simulink library "VIS_LIB"  (Simulink 8.6)
settings: Solver=ode45  StartTime=0.0  StopTime=10.0  RelTol=1e-3
undefined symbols (not defined in the file): AC, SIXOSEM_F_WD_AC_MASTER
libraries: cdsFilt x376, cdsEpicsOut x253, cdsEpicsIn x179, cdsTP x123, VIS_LIB x95, cdsMuxMatrix x91, cdsEpicsStringIn x75, cdsFiltCtrl x72, cdsFunctionCall x70, cdsRms x59, KAGRA_UTIL x25, STATE_BIO_MASTER x5
(part 6 of 38)

== system VIS_LIB/PReQua_3DOF ==
  Freq : Inport
  t : Inport  Port=2
  SampFreq : Inport  Port=3
  LEN_SIG : Inport  Port=4
  PIT_SIG : Inport  Port=5
  YAW_SIG1 : Inport  Port=6
  LEN_PHASE : Inport  Port=7
  PIT_PHASE : Inport  Port=8
  YAW_PHASE1 : Inport  Port=9
  Demux{1..6} (6 alike) : Demux  Outputs=3
  ENV_LEN : cdsFilt/Subsystem  Tag=cdsFilt  Description=|
      | Purpose:                                                                                                                                                                                                                                  
      | Standard CDS IIR filter module.                                                                                                                                                                                                           
      |                                                                                                                                                                                                                                           
      | Operation:                                                                                                                                                                                                                                
      | Consists of 10 second order section IIR filters, plus a ramped gain stage. In FE code, also provides pre-defined test points and excitation channel inputs. The filter coefficients are defined in the LIGO system using the 'foton' tool.
      |                                                                                                                                                                                                                                           
      | Usage:                                                                                                                                                                                                                                    
      | Name the part with the desired filter module name.
      settings: AttributesFormatString=%<Tag>
  ENV_PIT : cdsFilt/Subsystem  Tag=cdsFilt  Description=|
      | Purpose:                                                                                                                                                                                                                                  
      | Standard CDS IIR filter module.                                                                                                                                                                                                           
      |                                                                                                                                                                                                                                           
      | Operation:                                                                                                                                                                                                                                
      | Consists of 10 second order section IIR filters, plus a ramped gain stage. In FE code, also provides pre-defined test points and excitation channel inputs. The filter coefficients are defined in the LIGO system using the 'foton' tool.
      |                                                                                                                                                                                                                                           
      | Usage:                                                                                                                                                                                                                                    
      | Name the part with the desired filter module name.
      settings: AttributesFormatString=%<Tag>
  ENV_YAW : cdsFilt/Subsystem  Tag=cdsFilt  Description=|
      | Purpose:                                                                                                                                                                                                                                  
      | Standard CDS IIR filter module.                                                                                                                                                                                                           
      |                                                                                                                                                                                                                                           
      | Operation:                                                                                                                                                                                                                                
      | Consists of 10 second order section IIR filters, plus a ramped gain stage. In FE code, also provides pre-defined test points and excitation channel inputs. The filter coefficients are defined in the LIGO system using the 'foton' tool.
      |                                                                                                                                                                                                                                           
      | Usage:                                                                                                                                                                                                                                    
      | Name the part with the desired filter module name.
      settings: AttributesFormatString=%<Tag>
  LEN_CP : VIS_LIB/CALC_CP_COEF_3DOF
  Mux1 : Mux  Inputs=3
  Mux4 : Mux  Inputs=3
  PIT_CP : VIS_LIB/CALC_CP_COEF_3DOF
  QUALEN : KAGRA_UTIL/pReQua_ver2
  QUAPIT : KAGRA_UTIL/pReQua_ver2
  QUAYAW : KAGRA_UTIL/pReQua_ver2
  YAW_CP : VIS_LIB/CALC_CP_COEF_3DOF
  PhaseL : Outport
  PhaseP : Outport  Port=2
  PhaseY : Outport  Port=3
  wires:
  QUAPIT/1 -> ENV_PIT/1
  QUAPIT/2 -> PhaseP/1
  QUAYAW/1 -> ENV_YAW/1
  QUAYAW/2 -> PhaseY/1
  LEN_SIG/1 -> QUALEN/1
  LEN_PHASE/1 -> QUALEN/2
  PIT_SIG/1 -> QUAPIT/1
  PIT_PHASE/1 -> QUAPIT/2
  YAW_SIG1/1 -> QUAYAW/1
  YAW_PHASE1/1 -> QUAYAW/2
  Freq/1 -> Mux4/1
  t/1 -> Mux4/2
  SampFreq/1 -> Mux4/3
  Demux1/1 -> QUAPIT/3
  Demux1/2 -> QUAPIT/4
  Demux1/3 -> QUAPIT/5
  Demux2/1 -> QUAYAW/3
  Demux2/2 -> QUAYAW/4
  Demux2/3 -> QUAYAW/5
  Mux4/1 -> Demux1/1, Demux2/1, Demux6/1
  ENV_LEN/1 -> Mux1/1
  ENV_PIT/1 -> Mux1/2
  ENV_YAW/1 -> Mux1/3
  Demux3/2 -> LEN_CP/3
  Demux3/1 -> LEN_CP/1, LEN_CP/2
  Demux3/3 -> LEN_CP/4
  Demux4/1 -> PIT_CP/2
  Demux4/2 -> PIT_CP/1, PIT_CP/3
  Demux4/3 -> PIT_CP/4
  Demux5/1 -> YAW_CP/2
  Demux5/2 -> YAW_CP/3
  Demux5/3 -> YAW_CP/1, YAW_CP/4
  Mux1/1 -> Demux5/1, Demux4/1, Demux3/1
  Demux6/1 -> QUALEN/3
  Demux6/2 -> QUALEN/4
  Demux6/3 -> QUALEN/5
  QUALEN/2 -> PhaseL/1
  QUALEN/1 -> ENV_LEN/1

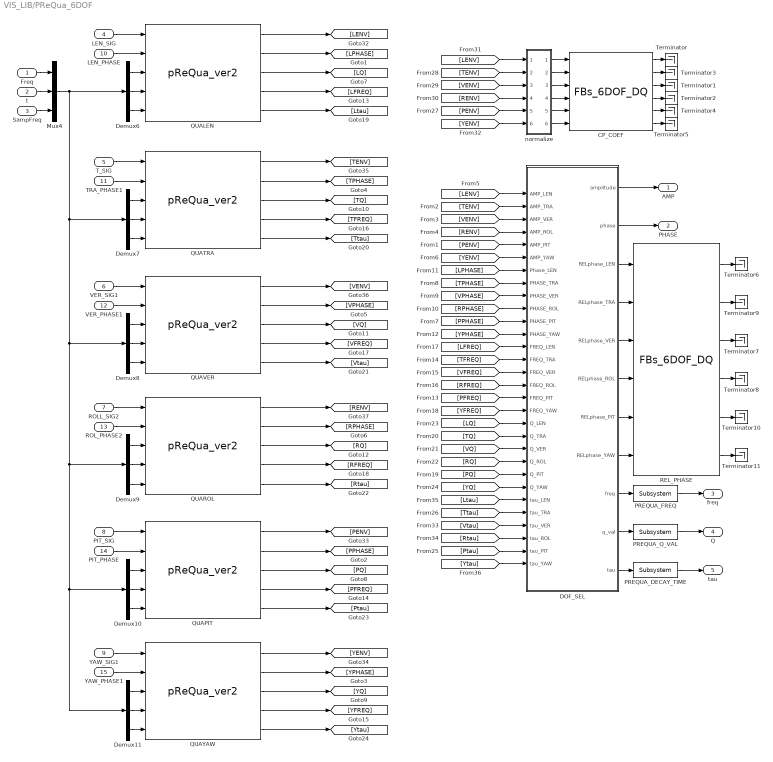
== system VIS_LIB/PReQua_6DOF ==
  Freq : Inport
  t : Inport  Port=2
  SampFreq : Inport  Port=3
  LEN_SIG : Inport  Port=4
  T_SIG : Inport  Port=5
  VER_SIG1 : Inport  Port=6
  ROLL_SIG2 : Inport  Port=7
  PIT_SIG : Inport  Port=8
  YAW_SIG1 : Inport  Port=9
  LEN_PHASE : Inport  Port=10
  TRA_PHASE1 : Inport  Port=11
  VER_PHASE1 : Inport  Port=12
  ROL_PHASE2 : Inport  Port=13
  PIT_PHASE : Inport  Port=14
  YAW_PHASE1 : Inport  Port=15
  CP_COEF : VIS_LIB/UTILs/FBs_6DOF_DQ
  DOF_SEL : Subsystem
  Demux{6..11} (6 alike) : Demux  Outputs=3
  Mux4 : Mux  Inputs=3
  PREQUA_DECAY_TIME : cdsFilt/Subsystem  Tag=cdsFilt  Description=|
      | Purpose:                                                                                                                                                                                                                                  
      | Standard CDS IIR filter module.                                                                                                                                                                                                           
      |                                                                                                                                                                                                                                           
      | Operation:                                                                                                                                                                                                                                
      | Consists of 10 second order section IIR filters, plus a ramped gain stage. In FE code, also provides pre-defined test points and excitation channel inputs. The filter coefficients are defined in the LIGO system using the 'foton' tool.
      |                                                                                                                                                                                                                                           
      | Usage:                                                                                                                                                                                                                                    
      | Name the part with the desired filter module name.
      settings: AttributesFormatString=%<Tag>
  PREQUA_FREQ : cdsFilt/Subsystem  Tag=cdsFilt  Description=|
      | Purpose:                                                                                                                                                                                                                                  
      | Standard CDS IIR filter module.                                                                                                                                                                                                           
      |                                                                                                                                                                                                                                           
      | Operation:                                                                                                                                                                                                                                
      | Consists of 10 second order section IIR filters, plus a ramped gain stage. In FE code, also provides pre-defined test points and excitation channel inputs. The filter coefficients are defined in the LIGO system using the 'foton' tool.
      |                                                                                                                                                                                                                                           
      | Usage:                                                                                                                                                                                                                                    
      | Name the part with the desired filter module name.
      settings: AttributesFormatString=%<Tag>
  PREQUA_Q_VAL : cdsFilt/Subsystem  Tag=cdsFilt  Description=|
      | Purpose:                                                                                                                                                                                                                                  
      | Standard CDS IIR filter module.                                                                                                                                                                                                           
      |                                                                                                                                                                                                                                           
      | Operation:                                                                                                                                                                                                                                
      | Consists of 10 second order section IIR filters, plus a ramped gain stage. In FE code, also provides pre-defined test points and excitation channel inputs. The filter coefficients are defined in the LIGO system using the 'foton' tool.
      |                                                                                                                                                                                                                                           
      | Usage:                                                                                                                                                                                                                                    
      | Name the part with the desired filter module name.
      settings: AttributesFormatString=%<Tag>
  QUALEN : KAGRA_UTIL/pReQua_ver2
  QUAPIT : KAGRA_UTIL/pReQua_ver2
  QUAROL : KAGRA_UTIL/pReQua_ver2
  QUATRA : KAGRA_UTIL/pReQua_ver2
  QUAVER : KAGRA_UTIL/pReQua_ver2
  QUAYAW : KAGRA_UTIL/pReQua_ver2
  REL_PHASE : VIS_LIB/UTILs/FBs_6DOF_DQ
  Terminator{,1..11} (12 alike) : Terminator
  normalize : Subsystem
  AMP : Outport
  PHASE : Outport  Port=2
  freq : Outport  Port=3
  Q : Outport  Port=4
  tau : Outport  Port=5
  wires:
  DOF_SEL/8(RELphase_YAW) -> REL_PHASE/6
  DOF_SEL/7(RELphase_PIT) -> REL_PHASE/5
  DOF_SEL/6(RELphase_ROL) -> REL_PHASE/4
  DOF_SEL/5(RELphase_VER) -> REL_PHASE/3
  DOF_SEL/4(RELphase_TRA) -> REL_PHASE/2
  DOF_SEL/3(RELphase_LEN) -> REL_PHASE/1
  PREQUA_DECAY_TIME/1 -> tau/1
  PREQUA_Q_VAL/1 -> Q/1
  PREQUA_FREQ/1 -> freq/1
  REL_PHASE/6 -> Terminator11/1
  REL_PHASE/5 -> Terminator10/1
  REL_PHASE/4 -> Terminator8/1
  REL_PHASE/3 -> Terminator7/1
  REL_PHASE/2 -> Terminator9/1
  REL_PHASE/1 -> Terminator6/1
  CP_COEF/6 -> Terminator5/1
  CP_COEF/5 -> Terminator4/1
  CP_COEF/4 -> Terminator2/1
  CP_COEF/3 -> Terminator1/1
  normalize/6(Out6) -> CP_COEF/6
  normalize/5(Out5) -> CP_COEF/5
  normalize/4(Out4) -> CP_COEF/4
  normalize/3(Out3) -> CP_COEF/3
  normalize/2(Out2) -> CP_COEF/2
  normalize/1(Out1) -> CP_COEF/1
  [Ytau] -> DOF_SEL/30(tau_YAW)
  [Ptau] -> DOF_SEL/29(tau_PIT)
  [Rtau] -> DOF_SEL/28(tau_ROL)
  [Vtau] -> DOF_SEL/27(tau_VER)
  [Ttau] -> DOF_SEL/26(tau_TRA)
  [Ltau] -> DOF_SEL/25(tau_LEN)
  DOF_SEL/11(tau) -> PREQUA_DECAY_TIME/1
  QUAPIT/5 -> [Ptau]
  QUAYAW/5 -> [Ytau]
  QUAVER/5 -> [Vtau]
  QUAROL/5 -> [Rtau]
  QUATRA/5 -> [Ttau]
  QUALEN/5 -> [Ltau]
  DOF_SEL/10(q_val) -> PREQUA_Q_VAL/1
  DOF_SEL/9(freq) -> PREQUA_FREQ/1
  QUALEN/4 -> [LFREQ]
  QUAPIT/4 -> [PFREQ]
  QUAYAW/4 -> [YFREQ]
  QUATRA/4 -> [TFREQ]
  QUAVER/4 -> [VFREQ]
  QUAROL/4 -> [RFREQ]
  QUALEN/3 -> [LQ]
  QUAPIT/3 -> [PQ]
  QUAYAW/3 -> [YQ]
  QUATRA/3 -> [TQ]
  QUAVER/3 -> [VQ]
  QUAROL/3 -> [RQ]
  [YQ] -> DOF_SEL/24(Q_YAW)
  [PQ] -> DOF_SEL/23(Q_PIT)
  [RQ] -> DOF_SEL/22(Q_ROL)
  [VQ] -> DOF_SEL/21(Q_VER)
  [TQ] -> DOF_SEL/20(Q_TRA)
  [LQ] -> DOF_SEL/19(Q_LEN)
  [YFREQ] -> DOF_SEL/18(FREQ_YAW)
  [PFREQ] -> DOF_SEL/17(FREQ_PIT)
  [RFREQ] -> DOF_SEL/16(FREQ_ROL)
  [VFREQ] -> DOF_SEL/15(FREQ_VER)
  [TFREQ] -> DOF_SEL/14(FREQ_TRA)
  [LFREQ] -> DOF_SEL/13(FREQ_LEN)
  DOF_SEL/2(phase) -> PHASE/1
  DOF_SEL/1(amplitude) -> AMP/1
  [YPHASE] -> DOF_SEL/12(PHASE_YAW)
  [PPHASE] -> DOF_SEL/11(PHASE_PIT)
  [RPHASE] -> DOF_SEL/10(PHASE_ROL)
  [VPHASE] -> DOF_SEL/9(PHASE_VER)
  [TPHASE] -> DOF_SEL/8(PHASE_TRA)
  [LPHASE] -> DOF_SEL/7(Phase_LEN)
  [YENV] -> DOF_SEL/6(AMP_YAW)
  [PENV] -> DOF_SEL/5(AMP_PIT)
  [RENV] -> DOF_SEL/4(AMP_ROL)
  [VENV] -> DOF_SEL/3(AMP_VER)
  [TENV] -> DOF_SEL/2(AMP_TRA)
  [LENV] -> DOF_SEL/1(AMP_LEN)
  QUALEN/2 -> [LPHASE]
  CP_COEF/2 -> Terminator3/1
  CP_COEF/1 -> Terminator/1
  QUAPIT/2 -> [PPHASE]
  QUAYAW/2 -> [YPHASE]
  QUAVER/2 -> [VPHASE]
  QUATRA/2 -> [TPHASE]
  QUAROL/2 -> [RPHASE]
  QUALEN/1 -> [LENV]
  QUAPIT/1 -> [PENV]
  QUAYAW/1 -> [YENV]
  QUATRA/1 -> [TENV]
  QUAVER/1 -> [VENV]
  QUAROL/1 -> [RENV]
  LEN_SIG/1 -> QUALEN/1
  LEN_PHASE/1 -> QUALEN/2
  T_SIG/1 -> QUATRA/1
  VER_SIG1/1 -> QUAVER/1
  YAW_SIG1/1 -> QUAYAW/1
  PIT_SIG/1 -> QUAPIT/1
  ROLL_SIG2/1 -> QUAROL/1
  YAW_PHASE1/1 -> QUAYAW/2
  PIT_PHASE/1 -> QUAPIT/2
  ROL_PHASE2/1 -> QUAROL/2
  VER_PHASE1/1 -> QUAVER/2
  TRA_PHASE1/1 -> QUATRA/2
  Demux6/1 -> QUALEN/3
  Demux6/2 -> QUALEN/4
  Demux6/3 -> QUALEN/5
  Freq/1 -> Mux4/1
  t/1 -> Mux4/2
  SampFreq/1 -> Mux4/3
  Demux7/1 -> QUATRA/3
  Demux7/2 -> QUATRA/4
  Demux7/3 -> QUATRA/5
  Demux8/1 -> QUAVER/3
  Demux8/2 -> QUAVER/4
  Demux8/3 -> QUAVER/5
  Demux9/1 -> QUAROL/3
  Demux9/2 -> QUAROL/4
  Demux9/3 -> QUAROL/5
  Demux10/1 -> QUAPIT/3
  Demux10/2 -> QUAPIT/4
  Demux10/3 -> QUAPIT/5
  Demux11/1 -> QUAYAW/3
  Demux11/2 -> QUAYAW/4
  Demux11/3 -> QUAYAW/5
  Mux4/1 -> Demux7/1, Demux8/1, Demux10/1, Demux11/1, Demux9/1, Demux6/1
  [LENV] -> normalize/1(In1)
  [TENV] -> normalize/2(In2)
  [VENV] -> normalize/3(In3)
  [RENV] -> normalize/4(In4)
  [PENV] -> normalize/5(In5)
  [YENV] -> normalize/6(In6)

== system VIS_LIB/QUAASC1 ==
  Freq : Inport
  t : Inport  Port=2
  SampFreq : Inport  Port=3
  P_SIG : Inport  Port=4
  Y_SIG : Inport  Port=5
  P_SIG2 : Inport  Port=6
  Y_SIG2 : Inport  Port=7
  P_PHASE1 : Inport  Port=8
  Y_PHASE1 : Inport  Port=9
  P_PHASE2 : Inport  Port=10
  Y_PHASE2 : Inport  Port=11
  CP_COEF : Subsystem
  DOF_SEL : Subsystem
  Demux{6..9} (4 alike) : Demux  Outputs=3
  ETM_PIT : KAGRA_UTIL/pReQua_ver2
  ETM_YAW : KAGRA_UTIL/pReQua_ver2
  ITM_PIT : KAGRA_UTIL/pReQua_ver2
  ITM_YAW : KAGRA_UTIL/pReQua_ver2
  Mux4 : Mux  Inputs=3
  REL_PHASE : Subsystem
  Terminator{,1..19} (20 alike) : Terminator
  normalize : Subsystem
  wires:
  CP_COEF/4(ROL_OUT) -> Terminator2/1
  CP_COEF/3(VER_OUT) -> Terminator1/1
  normalize/4(Out4) -> CP_COEF/4(ROL_IN)
  normalize/3(Out3) -> CP_COEF/3(VER_IN)
  normalize/2(Out2) -> CP_COEF/2(TRA_IN)
  normalize/1(Out1) -> CP_COEF/1(LEN_IN)
  CP_COEF/2(TRA_OUT) -> Terminator3/1
  CP_COEF/1(LEN_OUT) -> Terminator/1
  ITM_PIT/1 -> [ENVITMP]
  ITM_YAW/1 -> [ENVITMY]
  ETM_PIT/1 -> [ENVETMP]
  ETM_YAW/1 -> [ENVETMY]
  P_SIG/1 -> ITM_PIT/1
  P_PHASE1/1 -> ITM_PIT/2
  Y_SIG/1 -> ITM_YAW/1
  P_SIG2/1 -> ETM_PIT/1
  Y_SIG2/1 -> ETM_YAW/1
  Y_PHASE2/1 -> ETM_YAW/2
  P_PHASE2/1 -> ETM_PIT/2
  Y_PHASE1/1 -> ITM_YAW/2
  Demux6/1 -> ITM_PIT/3
  Demux6/2 -> ITM_PIT/4
  Demux6/3 -> ITM_PIT/5
  Freq/1 -> Mux4/1
  t/1 -> Mux4/2
  SampFreq/1 -> Mux4/3
  Demux7/1 -> ITM_YAW/3
  Demux7/2 -> ITM_YAW/4
  Demux7/3 -> ITM_YAW/5
  Demux8/1 -> ETM_PIT/3
  Demux8/2 -> ETM_PIT/4
  Demux8/3 -> ETM_PIT/5
  Demux9/1 -> ETM_YAW/3
  Demux9/2 -> ETM_YAW/4
  Demux9/3 -> ETM_YAW/5
  Mux4/1 -> Demux7/1, Demux8/1, Demux9/1, Demux6/1
  ITM_PIT/5 -> Terminator4/1
  ITM_PIT/4 -> Terminator5/1
  ITM_PIT/3 -> Terminator6/1
  ITM_YAW/5 -> Terminator8/1
  ITM_YAW/4 -> Terminator9/1
  ITM_YAW/3 -> Terminator10/1
  ETM_PIT/5 -> Terminator12/1
  ETM_PIT/4 -> Terminator13/1
  ETM_PIT/3 -> Terminator14/1
  ETM_YAW/5 -> Terminator16/1
  ETM_YAW/4 -> Terminator17/1
  ETM_YAW/3 -> Terminator18/1
  ITM_PIT/2 -> [PHITMP]
  ITM_YAW/2 -> [PHITMY]
  ETM_PIT/2 -> [PHETMP]
  ETM_YAW/2 -> [PHETMY]
  [ENVITMP] -> normalize/1(In1)
  [ENVITMY] -> normalize/2(In2)
  [ENVETMP] -> normalize/3(In3)
  [ENVETMY] -> normalize/4(In4)
  [PHITMP] -> DOF_SEL/1(Phase_LEN)
  [PHITMY] -> DOF_SEL/2(PHASE_TRA)
  [PHETMP] -> DOF_SEL/3(PHASE_VER)
  [PHETMY] -> DOF_SEL/4(PHASE_ROL)
  DOF_SEL/1(RELphase_LEN) -> REL_PHASE/1(LEN_IN)
  DOF_SEL/2(RELphase_TRA) -> REL_PHASE/2(TRA_IN)
  DOF_SEL/3(RELphase_VER) -> REL_PHASE/3(VER_IN)
  DOF_SEL/4(RELphase_ROL) -> REL_PHASE/4(ROL_IN)
  REL_PHASE/4(ROL_OUT) -> Terminator15/1
  REL_PHASE/3(VER_OUT) -> Terminator11/1
  REL_PHASE/2(TRA_OUT) -> Terminator19/1
  REL_PHASE/1(LEN_OUT) -> Terminator7/1

== system VIS_LIB/SHUTDOWN_TRIG_TYPEBP ==
  note: WDBLOCKFLAG is zero (0) if OK,
      | non-zero if BAD
  note: AND is zero  (0) if all stages are OK
      | non-zero if BAD
  SF_WDBLOCKFLAG_In : Inport
  BF_WDBLOCKFLAG_In : Inport  Port=2
  IM_WDBLOCKFLAG_In : Inport  Port=3
  TM_WDBLOCKFLAG_In : Inport  Port=4
  LogicalOperator1 : Logic  Operator=OR  Inputs=4  AllPortsSameDT=off  OutDataTypeStr=boolean
  STATE : cdsEpicsOut/Subsystem  Tag=cdsEpicsOutput  Description=|
      | Purpose:                                          
      | Output a FE signal to an EPICS channel.           
      |                                                   
      | Operation:                                        
      | Takes input value and passes it to EPICS record.  
      |                                                   
      | Usage:                                            
      | Name the part with the desired EPICS rrecord name.
      settings: AttributesFormatString=%<Tag>
  DACKILL_TRIG_Out : Outport
  wires:
  STATE/1 -> DACKILL_TRIG_Out/1
  LogicalOperator1/1 -> STATE/1
  SF_WDBLOCKFLAG_In/1 -> LogicalOperator1/1
  BF_WDBLOCKFLAG_In/1 -> LogicalOperator1/2
  IM_WDBLOCKFLAG_In/1 -> LogicalOperator1/3
  TM_WDBLOCKFLAG_In/1 -> LogicalOperator1/4

== system VIS_LIB/UTILs ==
  1COIL_DQ : Subsystem
  3COILs : Subsystem
  3COILs_DQ : Subsystem
  4COILs : Subsystem
  4COILs_DQ : Subsystem
  4SEG_DQ : Subsystem
  6COILs : Subsystem
  6COILs_DQ : Subsystem
  7COILs_DQ1 : Subsystem
  DRIVEALIGN : Subsystem
  FBs_2DOF : Subsystem
  FBs_2DOF_DQ : Subsystem
  FBs_3DOF : Subsystem
  FBs_3DOF_DQ : Subsystem
  FBs_3DOF_IP : Subsystem
  FBs_3DOF_IP_DQ : Subsystem
  FBs_5STAGE : Subsystem
  FBs_5STAGE_DQ : Subsystem
  FBs_6DOF : Subsystem
  FBs_6DOF_DQ : Subsystem
  OL : Subsystem
  PAY_6DoF : Subsystem
  PAY_6DoF_DQ : Subsystem
  PAY_COILs_DQ : Subsystem

== system VIS_LIB/WD ==
  OSEM_UL_In : Inport
  OSEM_LL_In : Inport  Port=2
  OSEM_UR_In : Inport  Port=3
  OSEM_LR_In : Inport  Port=4
  ACT_UL_In : Inport  Port=5
  ACT_LL_In : Inport  Port=6
  ACT_UR_In : Inport  Port=7
  ACT_LR_In : Inport  Port=8
  ACT : FOUROSEM_WD_AC_MASTER/OSEMAC
  Ground5 : Ground
  OSEMAC : FOUROSEM_WD_AC_MASTER/OSEMAC
  OSEMDC : FOUROSEM_WD_DC_MASTER/OSEMDC
  RSET : cdsEpicsMomentary/EpicsMomentary  Tag=cdsEpicsMomentary
      settings: AttributesFormatString=%<Tag>
  RESET_Out : Outport
  OSEM_DC_FLAG_Out : Outport  Port=2
  OSEM_AC_FLAG_Out : Outport  Port=3
  ACT_FLAG_Out : Outport  Port=4
  wires:
  ACT/1 -> ACT_FLAG_Out/1
  ACT_LR_In/1 -> ACT/4
  ACT_UR_In/1 -> ACT/3
  OSEMAC/1 -> OSEM_AC_FLAG_Out/1
  RSET/1 -> RESET_Out/1
  OSEMDC/1 -> OSEM_DC_FLAG_Out/1
  Ground5/1 -> RSET/1
  ACT_LL_In/1 -> ACT/2
  ACT_UL_In/1 -> ACT/1
  OSEM_UL_In/1 -> OSEMDC/1, OSEMAC/1
  OSEM_LL_In/1 -> OSEMDC/2, OSEMAC/2
  OSEM_UR_In/1 -> OSEMDC/3, OSEMAC/3
  OSEM_LR_In/1 -> OSEMDC/4, OSEMAC/4

== system VIS_LIB/WD1 ==
  OSEM_H1_In : Inport
  OSEM_H2_In : Inport  Port=2
  OSEM_H3_In : Inport  Port=3
  OSEM_H4_In : Inport  Port=4
  OSEMAC : FOUROSEM_WD_AC_MASTER/OSEMAC
  OSEM_AC_FLAG_Out : Outport
  wires:
  OSEMAC/1 -> OSEM_AC_FLAG_Out/1
  OSEM_H1_In/1 -> OSEMAC/1
  OSEM_H3_In/1 -> OSEMAC/3
  OSEM_H2_In/1 -> OSEMAC/2
  OSEM_H4_In/1 -> OSEMAC/4

== system VIS_LIB/WD2 ==
  LVDT_F0_In : Inport
  LVDT_SF_In : Inport  Port=2
  LVDT_BF_In : Inport  Port=3
  AC : Subsystem
  LVDT_AC_FLAG_Out : Outport
  wires:
  AC/1(FLAG) -> LVDT_AC_FLAG_Out/1
  LVDT_BF_In/1 -> AC/3(BF_In)
  LVDT_SF_In/1 -> AC/2(SF_In)
  LVDT_F0_In/1 -> AC/1(F0_In)

== system VIS_LIB/WD3 ==
  OSEM_V1_In : Inport
  OSEM_V2_In : Inport  Port=2
  OSEM_V3_In : Inport  Port=3
  OSEM_H1_In : Inport  Port=4
  OSEM_H2_In : Inport  Port=5
  OSEM_H3_In : Inport  Port=6
  OSEMAC : Subsystem  AncestorBlock=SIXOSEM_F_WD_AC_MASTER/AC
  OSEM_AC_FLAG_Out : Outport
  wires:
  OSEMAC/1(FLAG) -> OSEM_AC_FLAG_Out/1
  OSEM_V1_In/1 -> OSEMAC/1(V1_In)
  OSEM_V2_In/1 -> OSEMAC/2(V2_In)
  OSEM_V3_In/1 -> OSEMAC/3(V3_In)
  OSEM_H1_In/1 -> OSEMAC/4(H1_In)
  OSEM_H2_In/1 -> OSEMAC/5(H2_In1)
  OSEM_H3_In/1 -> OSEMAC/6(H3_In1)

== system VIS_LIB/WD4 ==
  LVDT_SF_In : Inport
  LVDT_BF_In : Inport  Port=2
  AC : Subsystem
  LVDT_AC_FLAG_Out : Outport
  wires:
  AC/1(FLAG) -> LVDT_AC_FLAG_Out/1
  LVDT_BF_In/1 -> AC/2(BF_In)
  LVDT_SF_In/1 -> AC/1(SF_In)

== system VIS_LIB/WDMON ==
  BLOCK_Flag : Inport
  STATE_Flag : Inport  Port=2
  FIRST_Flag : Inport  Port=3
  CURRENT_Flag : Inport  Port=4
  BLOCK : cdsEpicsOut/Subsystem  Tag=cdsEpicsOutput  Description="field(PREC,\"3\")"
      settings: AttributesFormatString=%<Tag>
  CURRENTTRIG : cdsEpicsOut/Subsystem  Tag=cdsEpicsOutput  Description="field(PREC,\"3\")"
      settings: AttributesFormatString=%<Tag>
  FIRSTTRIG : cdsEpicsOut/Subsystem  Tag=cdsEpicsOutput  Description="field(PREC,\"3\")"
      settings: AttributesFormatString=%<Tag>
  STATE : cdsEpicsOut/Subsystem  Tag=cdsEpicsOutput  Description="field(PREC,\"3\")"
      settings: AttributesFormatString=%<Tag>
  Terminator{1,3,10..11} (4 alike) : Terminator
  wires:
  STATE_Flag/1 -> STATE/1
  FIRST_Flag/1 -> FIRSTTRIG/1
  CURRENT_Flag/1 -> CURRENTTRIG/1
  CURRENTTRIG/1 -> Terminator11/1
  FIRSTTRIG/1 -> Terminator10/1
  BLOCK_Flag/1 -> BLOCK/1
  BLOCK/1 -> Terminator1/1
  STATE/1 -> Terminator3/1

== system VIS_LIB/WD_BF ==
  LVDT_GAS_In : Inport
  LVDT_V1_In : Inport  Port=2
  LVDT_V2_In : Inport  Port=3
  LVDT_V3_In : Inport  Port=4
  LVDT_H1_In : Inport  Port=5
  LVDT_H2_In : Inport  Port=6
  LVDT_H3_In : Inport  Port=7
  AC : BF_WD_MASTER/AC
  AC_FLAG_Out : Outport
  wires:
  AC/1 -> AC_FLAG_Out/1
  LVDT_GAS_In/1 -> AC/1
  LVDT_V1_In/1 -> AC/2
  LVDT_V2_In/1 -> AC/3
  LVDT_V3_In/1 -> AC/4
  LVDT_H1_In/1 -> AC/5
  LVDT_H2_In/1 -> AC/6
  LVDT_H3_In/1 -> AC/7

== system VIS_LIB/WD_GAS ==
  GAS_In : Inport
  AC : GAS_WD_MASTER/GASAC
  GAS_AC_FLAG_Out : Outport
  wires:
  AC/1 -> GAS_AC_FLAG_Out/1
  GAS_In/1 -> AC/1

== system VIS_LIB/WD_TEST4CH ==
  SEN1_In : Inport
  SEN2_In : Inport  Port=2
  SEN3_In : Inport  Port=3
  SEN4_In : Inport  Port=4
  OSEMAC : FOUROSEM_WD_AC_MASTER/OSEMAC
  TESTSEN_AC_FLAG_Out : Outport
  wires:
  OSEMAC/1 -> TESTSEN_AC_FLAG_Out/1
  SEN1_In/1 -> OSEMAC/1
  SEN3_In/1 -> OSEMAC/3
  SEN2_In/1 -> OSEMAC/2
  SEN4_In/1 -> OSEMAC/4
